simulink model "Library"  (Simulink 7.7)
settings: Solver=ode45  StartTime=0.0  StopTime=10.0  RelTol=1e-3
undefined symbols (not defined in the file or in its folder): quad
settings Model: Creator=Alexey  LastModifiedBy=Alexey

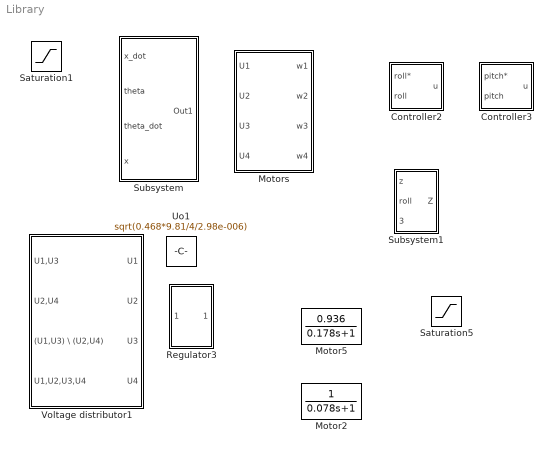
== system Library ==
  Controller2 : Subsystem
  Controller3 : Subsystem
  Motor2 : TransferFcn  Denominator=[0.078 1]
  Motor5 : TransferFcn  Numerator=[0.936]  Denominator=[0.178 1]
  Motors : Subsystem
  Regulator3 : Subsystem
  Saturation1 : Saturate  UpperLimit=10*pi/180  LowerLimit=-10*pi/180
  Saturation5 : Saturate  UpperLimit=700  LowerLimit=150
  Subsystem : Subsystem
  Subsystem1 : Subsystem
  Uo1 : Constant  Value=sqrt(0.468*9.81/4/2.98e-006)
  Voltage distributor1 : Subsystem

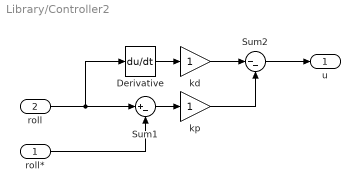
== system Library/Controller2 ==
  roll* : Inport
  roll : Inport  Port=2
  Derivative : Derivative
  Sum1 : Sum  Inputs=|+-
  Sum2 : Sum  Inputs=|--
  kd : Gain
  kp : Gain
  u : Outport
  wires:
  roll/1 -> Derivative/1, Sum1/1
  Sum1/1 -> kp/1
  roll*/1 -> Sum1/2
  Derivative/1 -> kd/1
  kd/1 -> Sum2/1
  kp/1 -> Sum2/2
  Sum2/1 -> u/1

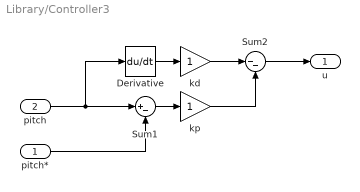
== system Library/Controller3 ==
  pitch* : Inport
  pitch : Inport  Port=2
  Derivative : Derivative
  Sum1 : Sum  Inputs=|+-
  Sum2 : Sum  Inputs=|--
  kd : Gain
  kp : Gain
  u : Outport
  wires:
  pitch/1 -> Derivative/1, Sum1/1
  Sum1/1 -> kp/1
  pitch*/1 -> Sum1/2
  Derivative/1 -> kd/1
  kd/1 -> Sum2/1
  kp/1 -> Sum2/2
  Sum2/1 -> u/1

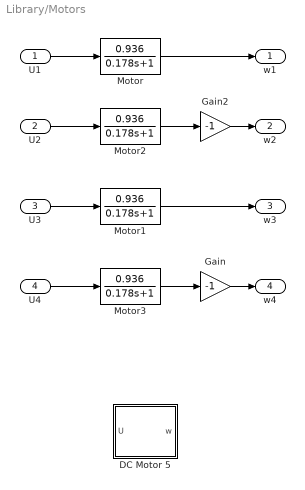
== system Library/Motors ==
  U1 : Inport
  U2 : Inport  Port=2
  U3 : Inport  Port=3
  U4 : Inport  Port=4
  DC Motor 5 : Subsystem
  Gain : Gain  Gain=-1
  Gain2 : Gain  Gain=-1
  Motor{,1..3} (4 alike) : TransferFcn  Numerator=[0.936]  Denominator=[0.178 1]
  w1 : Outport
  w2 : Outport  Port=2
  w3 : Outport  Port=3
  w4 : Outport  Port=4
  wires:
  U1/1 -> Motor/1
  Motor/1 -> w1/1
  U3/1 -> Motor1/1
  U2/1 -> Motor2/1
  Motor2/1 -> Gain2/1
  Motor1/1 -> w3/1
  Motor3/1 -> Gain/1
  U4/1 -> Motor3/1
  Gain/1 -> w4/1
  Gain2/1 -> w2/1

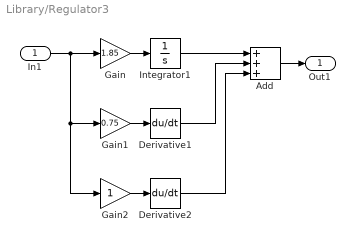
== system Library/Regulator3 ==
  In1 : Inport
  Add : Sum  Inputs=+++
  Derivative1 : Derivative
  Derivative2 : Derivative
  Gain : Gain  Gain=1.85
  Gain1 : Gain  Gain=0.75
  Gain2 : Gain
  Integrator1 : Integrator
  Out1 : Outport
  wires:
  Add/1 -> Out1/1
  In1/1 -> Gain2/1, Gain1/1, Gain/1
  Derivative2/1 -> Add/3
  Derivative1/1 -> Add/2
  Integrator1/1 -> Add/1
  Gain1/1 -> Derivative1/1
  Gain2/1 -> Derivative2/1
  Gain/1 -> Integrator1/1

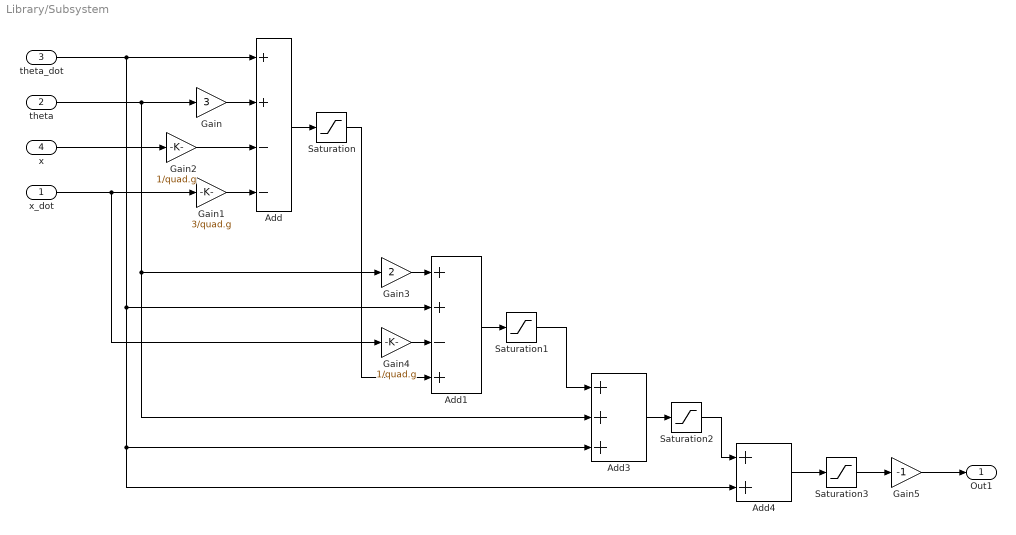
== system Library/Subsystem ==
  x_dot : Inport
  theta : Inport  Port=2
  theta_dot : Inport  Port=3
  x : Inport  Port=4
  Add : Sum  Inputs=++--
  Add1 : Sum  Inputs=++-+
  Add3 : Sum  Inputs=+++
  Add4 : Sum
  Gain : Gain  Gain=3
  Gain1 : Gain  Gain=3/quad.g
  Gain2 : Gain  Gain=1/quad.g
  Gain3 : Gain  Gain=2
  Gain4 : Gain  Gain=1/quad.g
  Gain5 : Gain  Gain=-1
  Saturation{,1..3} (4 alike) : Saturate
  Out1 : Outport
  wires:
  Gain3/1 -> Add1/1
  Gain4/1 -> Add1/3
  Gain/1 -> Add/2
  Gain2/1 -> Add/3
  Gain1/1 -> Add/4
  Add/1 -> Saturation/1
  theta_dot/1 -> Add/1, Add1/2, Add3/3, Add4/2
  theta/1 -> Gain/1, Gain3/1, Add3/2
  x/1 -> Gain2/1
  x_dot/1 -> Gain1/1, Gain4/1
  Saturation/1 -> Add1/4
  Add1/1 -> Saturation1/1
  Saturation1/1 -> Add3/1
  Add3/1 -> Saturation2/1
  Saturation2/1 -> Add4/1
  Add4/1 -> Saturation3/1
  Saturation3/1 -> Gain5/1
  Gain5/1 -> Out1/1

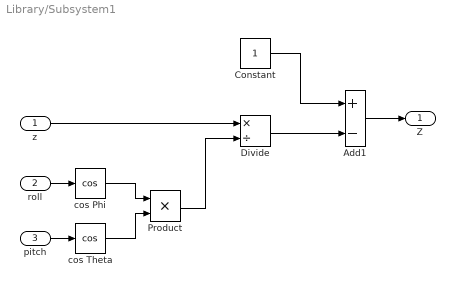
== system Library/Subsystem1 ==
  z : Inport
  roll : Inport  Port=2
  pitch : Inport  Port=3
  Add1 : Sum  Inputs=+-
  Constant : Constant
  Divide : Product  Inputs=*/
  Product : Product  RndMeth=Zero
  cos Phi : Trigonometry  Operator=cos
  cos Theta : Trigonometry  Operator=cos
  Z : Outport
  wires:
  cos Phi/1 -> Product/1
  cos Theta/1 -> Product/2
  Product/1 -> Divide/2
  Constant/1 -> Add1/1
  Divide/1 -> Add1/2
  Add1/1 -> Z/1
  z/1 -> Divide/1
  roll/1 -> cos Phi/1
  pitch/1 -> cos Theta/1

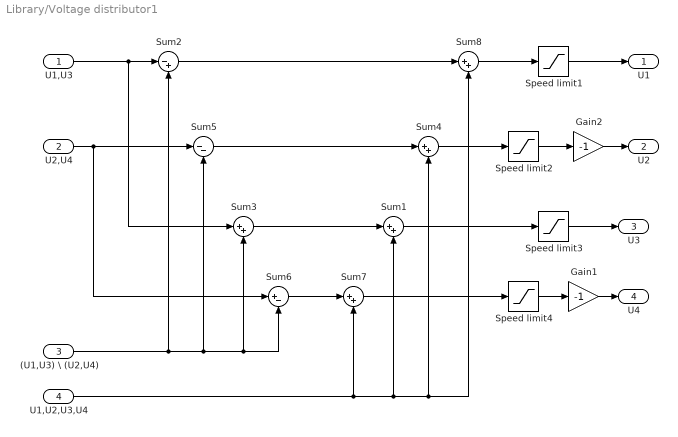
== system Library/Voltage distributor1 ==
  U1,U3 : Inport
  U2,U4 : Inport  Port=2
  (U1,U3) \ (U2,U4) : Inport  Port=3
  U1,U2,U3,U4 : Inport  Port=4
  Gain1 : Gain  Gain=-1
  Gain2 : Gain  Gain=-1
  Speed limit{1..4} (4 alike) : Saturate  UpperLimit=650  LowerLimit=550  ZeroCross=off
  Sum{1,4,7..8} (4 alike) : Sum  Inputs=|++
  Sum2 : Sum  Inputs=|-+
  Sum3 : Sum  Inputs=|++  SaturateOnIntegerOverflow=on  InputSameDT=on  OutDataTypeStr=Inherit: Same as first input
  Sum5 : Sum  Inputs=|--
  Sum6 : Sum  Inputs=|+-
  U1 : Outport
  U2 : Outport  Port=2
  U3 : Outport  Port=3
  U4 : Outport  Port=4
  wires:
  Gain1/1 -> U4/1
  Gain2/1 -> U2/1
  Speed limit4/1 -> Gain1/1
  Speed limit3/1 -> U3/1
  Speed limit2/1 -> Gain2/1
  Speed limit1/1 -> U1/1
  Sum7/1 -> Speed limit4/1
  Sum1/1 -> Speed limit3/1
  Sum4/1 -> Speed limit2/1
  Sum8/1 -> Speed limit1/1
  U1,U2,U3,U4/1 -> Sum8/2, Sum4/2, Sum1/2, Sum7/2
  Sum2/1 -> Sum8/1
  Sum5/1 -> Sum4/1
  Sum3/1 -> Sum1/1
  Sum6/1 -> Sum7/1
  (U1,U3) \ (U2,U4)/1 -> Sum5/2, Sum3/2, Sum6/2, Sum2/2
  U2,U4/1 -> Sum5/1, Sum6/1
  U1,U3/1 -> Sum3/1, Sum2/1

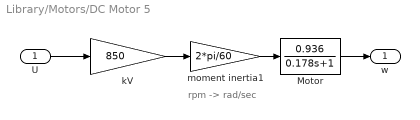
== system Library/Motors/DC Motor 5 ==
  note: rpm -> rad/sec
  U : Inport
  Motor : TransferFcn  Numerator=[0.936]  Denominator=[0.178 1]
  kV : Gain  Gain=850
  moment inertia1 : Gain  Gain=2*pi/60
  w : Outport
  wires:
  Motor/1 -> w/1
  moment inertia1/1 -> Motor/1
  kV/1 -> moment inertia1/1
  U/1 -> kV/1
